simulink model "simulering2"  (R2017a)
settings: Solver=VariableStepAuto  StartTime=0.0  StopTime=80.0  RelTol=1e-3
values from neighbouring files (symbols this model uses):
  Ad = 0.926549818887    [sysd.mat]    (also in trock.m = sysd.A)
  Bd = [-0.0657631580404 -0.00735568538738]    [sysd.mat]    (also in trock.m = [ sysd.B(5) sysd.B(6) ])
  Cd = [0.0055555252792 0.00510059552972]    [sysd.mat]    (also in trock.m = [ sysd.C(2); sysd.C(4) ])
  Dd = [-0.661477669827  -0.229336546845; -0.607310717919  -0.249936400478]    [sysd.mat]    (also in trock.m = [ sysd.D(2,5) sysd.D(2,6); sysd.D(4,5) sysd.D(4,6) ])
  Ed = [ sysd.B(2) sysd.B(4)]    [trock.m]
  Kd = [ sysd.D(2,2) sysd.D(2,4); sysd.D(4,2) sysd.D(4,4) ]    [trock.m]
  Ts = 0.1    [sysd.mat]    (also in trock.m = 600)
undefined symbols (not defined in the file or in its folder): DiscIntNeverNeededParam
settings Model: Creator=nvink  LastModifiedBy=nvink

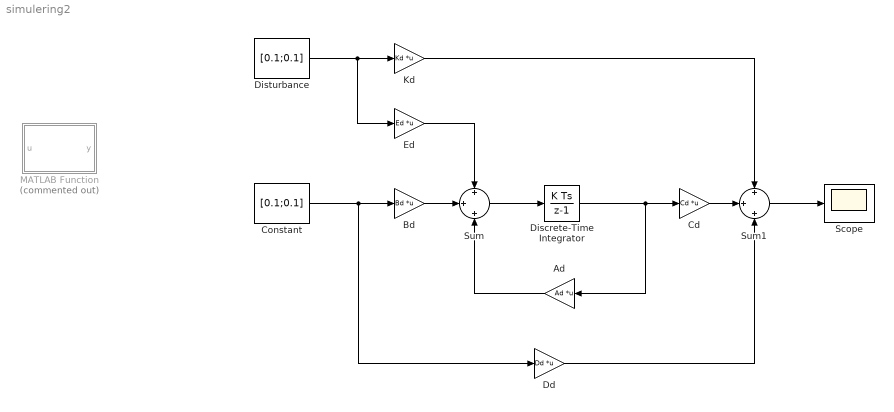
== system simulering2 ==
  Ad : Gain  Gain=Ad  Multiplication=Matrix(K*u)
  Bd : Gain  Gain=Bd  Multiplication=Matrix(K*u)
  "Cd " : Gain  Gain=Cd  Multiplication=Matrix(K*u)
  Constant : Constant  Value=[0.1;0.1]
  Dd : Gain  Gain=Dd  Multiplication=Matrix(K*u)
  Discrete-Time Integrator : DiscreteIntegrator  SampleTime=Ts  ICPrevOutput=DiscIntNeverNeededParam  ICPrevScaledInput=DiscIntNeverNeededParam
  Disturbance : Constant  Value=[0.1;0.1]
  Ed : Gain  Gain=Ed  Multiplication=Matrix(K*u)
  Kd : Gain  Gain=Kd  Multiplication=Matrix(K*u)
  MATLAB Function : MATLAB Function  Commented=on  TreatAsAtomicUnit=on
  Scope : Scope
  Sum : Sum  Inputs=+|+|+
  Sum1 : Sum  Inputs=+|+|+
  wires:
  Discrete-Time Integrator/1 -> Ad/1, "Cd "/1
  "Cd "/1 -> Sum1/2
  Bd/1 -> Sum/2
  Sum/1 -> Discrete-Time Integrator/1
  Ad/1 -> Sum/3
  Ed/1 -> Sum/1
  Disturbance/1 -> Kd/1, Ed/1
  Kd/1 -> Sum1/1
  Dd/1 -> Sum1/3
  Constant/1 -> Dd/1, Bd/1
  Sum1/1 -> Scope/1

== matlab function simulering2/MATLAB Function ==
  data: u input; y output
function y = fcn(u)
%%
%Solve a quadratic programming problem

%Variabels that we need to sort out.
% delta_p_0 d_hp U_bar_hp q_bar_p_hp

% Variabels that we use in the Matrix_op.m file
% Lambda_A Lambda_B Lambda_C Gamma Psi Phi Theta Omega Pi 
Matrix_op;
trock;                  %Load system matrices

delta_p_0 = 0.05;      %small-signal initial WT pressure measurement

d_hp = 0.05*90*ones(48,1);      % Small signal deviation of the Valves OD
U_bar_hp = 0.2*ones(48,1);      % Input pressure to ring pumps operating point
q_bar_p_hp = 1.4*ones(48,1);    % Flow operating point of the ring pumps

%%%%%%%%%%%%%%%%%% Generel QP %%%%%%%%%%%%%%%%%%
% 0.5*x'R*x+f'*x
%%%%%%%%%%%%%%%%%%%%%%%%%%%%%%%%%%%%%%%%%%%%%%%%%%%%%%%
%%%%%%%%%%%%%%%%%%%%% Constraint %%%%%%%%%%%%%%%%%%%%%%
%%%%%%%%%%%%%%%%%%%%%%%%%%%%%%%%%%%%%%%%%%%%%%%%%%%%%%%

% Output constraint
y_low =  0.08*ones(48,1);         % Full-signal upper and lower bounds 
y_high = 0.18*ones(48,1);           

% Pressure operating point of the PMA end-users
y_bar = [0.1562; 0.0991 ;0.1562; 0.0991 ;0.1562; 0.0991 ;0.1562; 0.0991 ;0.1562; 0.0991 ;0.1562; 0.0991 ;
        0.1562; 0.0991 ;0.1562; 0.0991 ;0.1562; 0.0991 ;0.1562; 0.0991 ;0.1562; 0.0991 ;0.1562; 0.0991 ;
        0.1562; 0.0991 ;0.1562; 0.0991 ;0.1562; 0.0991 ;0.1562; 0.0991 ;0.1562; 0.0991 ;0.1562; 0.0991 ;
        0.1562; 0.0991 ;0.1562; 0.0991 ;0.1562; 0.0991 ;0.1562; 0.0991 ;0.1562; 0.0991 ;0.1562; 0.0991];    

y1 = y_low - y_bar - Theta*Phi*delta_p_0-(Theta*Psi+Pi)*d_hp;
y2 = y_high - y_bar - Theta*Phi*delta_p_0-(Theta*Psi+Pi)*d_hp;
L_y = Theta*Gamma+Omega;

% State constraint
x_low = 0.055*ones(24,1);
x_high = 0.164*ones(24,1);
x_bar = 0.127*ones(24,1);

delta_p_wt_1 = x_low-x_bar - Phi*delta_p_0 - Psi*d_hp;
delta_p_wt_2 = x_high-x_bar - Phi*delta_p_0 - Psi*d_hp;

% input constraint 
u_low = -0.2;
u_high = 1;

%%%%%%%%%%%%%%%%%%%%%%%%%%%%%%%%%%%%%%%%%%%%%%%%%%%%%%%
%%%%%%%%%%%%%%%%%% Setting up the QP %%%%%%%%%%%%%%%%%% 
%%%%%%%%%%%%%%%%%%%%%%%%%%%%%%%%%%%%%%%%%%%%%%%%%%%%%%%

R = 2*(Lambda_A + Lambda_C*Gamma); 
R1=(R+R')/2;
R2=(R-R')/2;
f = U_bar_hp'*(Lambda_A+Lambda_C*Gamma)+d_hp'*(Lambda_B+Lambda_C*Psi)'+delta_p_0*(Lambda_C*Phi)'+q_bar_p_hp';

%CONSTRAINTS FOR Y AND X
A = [-L_y; L_y; -Gamma; Gamma];
b = [y1; y2; delta_p_wt_1; delta_p_wt_2];

%CONSTRAINTS only FOR Y
% A = [-L_y; L_y];
% b = [y1; y2];

%CONSTRAINTS only FOR X
% A = [-Gamma;Gamma];
% b = [delta_p_wt_1; delta_p_wt_2];

lb = u_low*ones(48,1);
ub = u_high*ones(48,1);

options = optimoptions('quadprog','Algorithm','interior-point-convex','Display','iter-detailed')
[u_hp,fval,exitflag,output,lambda] = quadprog(R1,f,[],[],[],[],lb,ub,[],options);

%fval,lambda
u_hp,exitflag,output

y = u_hp;
